simulink model "sgMdl_IO203_DigitalLoopback"  (R2024b)
settings: Solver=FixedStepAuto  StartTime=0.0  StopTime=inf  RelTol=1e-3  EnableMultiTasking=on
libraries: speedgoatlib_IO203 x3
Description:
  | IO203 - Digital Loopback
settings Model: ModifiedByFormat=Speedgoat  Creator=Speedgoat  LastModifiedBy=Speedgoat
settings SolverCC: ConcurrentTasks=on  AlgebraicLoopSolver=TrustRegion  PositivePriorityOrder=on
settings DataIOCC: LimitDataPoints=on  SaveFormat=Array  SignalLoggingSaveFormat=ModelDataLogs  ReturnWorkspaceOutputs=off
settings OptimizationCC: BlockReduction=off  OptimizeBlockIOStorage=off  BufferReuse=off  ReuseModelBlockBuffer=off  GlobalBufferReuse=off  ExpressionFolding=off  ExpressionDepthLimit=2147483647  LocalBlockOutputs=off
settings DebuggingCC: UnderspecifiedInitializationDetection=Classic  MergeDetectMultiDrivingBlocksExec=none  SolverPrmCheckMsg=warning  TasksWithSamePriorityMsg=none  FcnCallInpInsideContextMsg=warning  StateNameClashWarn=warning  SFUnexpectedBacktrackingDiag=warning  SFNoUnconditionalDefaultTransitionDiag=warning  SFExecutionAtInitializationDiag=none  ArithmeticOperatorsInVariantConditions=warning
settings HardwareCC: ProdBitPerLong=64  ProdLongLongMode=on  ProdHWDeviceType=Intel->x86-64 (Linux 64)
settings ModelReferenceCC: EnableRefExpFcnMdlSchedulingChecks=on  PropagateSignalLabelsOutOfModel=off
settings SFSimCC: SimUseLocalCustomCode=off  CustomCodeUndefinedFunction=UseInterfaceOnly
settings RTWCC: Description=Speedgoat Real-Time Target Machine  SystemTargetFile=speedgoat.tlc  TemplateMakefile=slrealtime_default_tmf  RTWUseLocalCustomCode=off  Toolchain=Simulink Real-Time Toolchain  BuildConfiguration=Faster Runs  TargetLang=C++  GPUComputeCapability=3.5  DLArmComputeVersion=19.05
settings CodeAppCC: StateflowObjectComments=on
settings SimulinkRealTimeTargetCC: SubcomponentCodeInterfacePackaging=Reusable function  InstructionSetFMA=off  LogToMDFFile=off  SLRTFileLogMaxRuns=10
settings ConfigComp: CovMetricSettings=dw  CovSaveCumulativeToWorkspaceVar=on  CovSaveSingleToWorkspaceVar=on  CovExternalEMLEnable=off  CovSFcnEnable=off  CovBoundaryAbsTol=1.0e-5

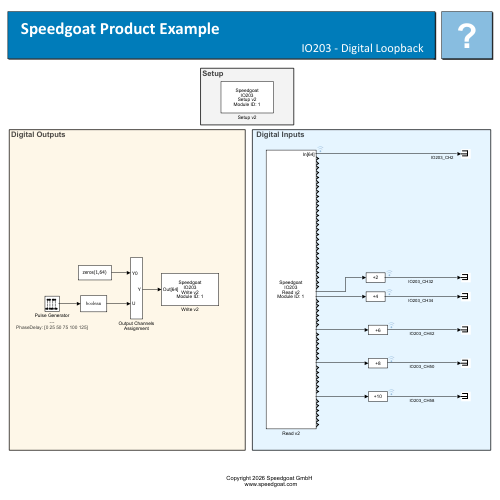
[thumbnail: Simulink's stored preview of the top-level diagram]
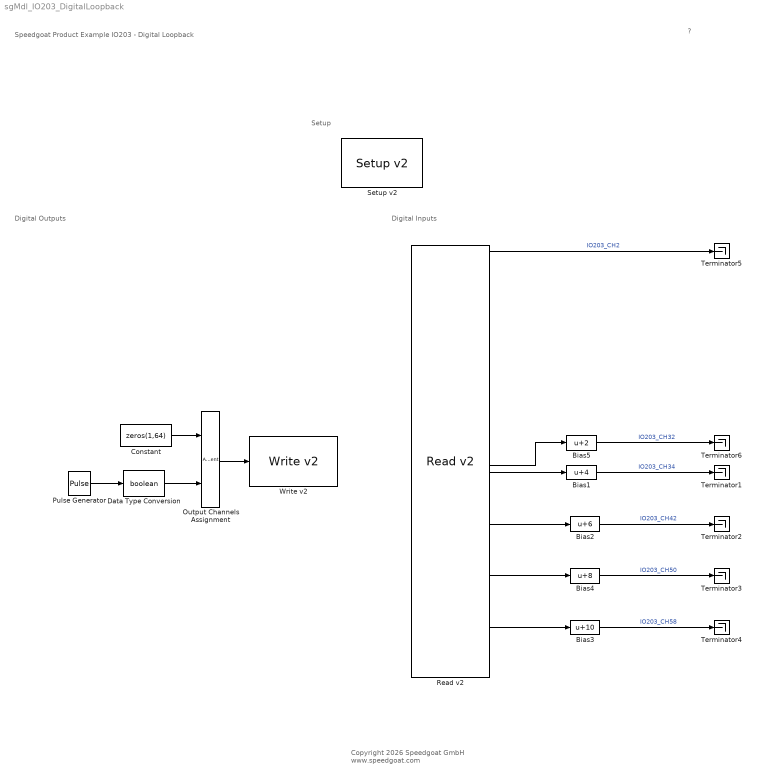
== system sgMdl_IO203_DigitalLoopback ==
  note: Digital Outputs
  note: Setup
  note: Digital Inputs
  note: Speedgoat Product Example
      | IO203 - Digital Loopback
  note: ?
  note: Copyright 2026 Speedgoat GmbH
      |  www.speedgoat.com
  Bias1 : Bias  Bias=4  SaturateOnIntegerOverflow=off
  Bias2 : Bias  Bias=6  SaturateOnIntegerOverflow=off
  Bias3 : Bias  Bias=10  SaturateOnIntegerOverflow=off
  Bias4 : Bias  Bias=8  SaturateOnIntegerOverflow=off
  Bias5 : Bias  Bias=2  SaturateOnIntegerOverflow=off
  Constant : Constant  Value=zeros(1,64)  OutDataTypeStr=boolean  SampleTime=-1
  Data Type Conversion : DataTypeConversion  OutDataTypeStr=boolean  SaturateOnIntegerOverflow=off  RndMeth=Floor
  Output Channels Assignment : Assignment  DiagnosticForDimensions=Warning  IndexOptions=Index vector (dialog)  Indices=[1 31 33 41 49 57]  OutputSizes=1
  Pulse Generator : DiscretePulseGenerator  Period=[100 100 100 200 200 200]  PulseWidth=[50 50 50 100 100 100]  PhaseDelay=[0 25 50 75 100 125]  SampleTime=0.001
      settings: AttributesFormatString=|
      | ---
      | PhaseDelay: %<PhaseDelay>
  Read v2 : speedgoatlib_IO203/Read v2   parId=1  parPortConf=1 port for each active input channel  parDataType=Double  parSampleTime=0.001  readPorts=[2 3 4 5 6 7 8 9 10 11 12 13 14 15 16 17 18 19 20 21 22 23 24 25 26 27 28 29 30 32 34 35 36 37 38 39 40 42 43 44 45 46 47 48 50 51 52 53 54 55 56 58 59 60 61 62 63 64]  portList=[2 3 4 5 6 7 8 9 10 11 12 13 14 15 16 17 18 19 20 21 22 23 24 25 26 27 28 29 30 32 34 35 36 37 38 39 40 42 43 44 45 46 47 48 50 51 52 53 54 55 56 58 59 60 61 62 63 64]  parPciSlot=-1  parNumOfPorts=58
      settings: SourceProductName=IO203
  Setup v2 : speedgoatlib_IO203/Setup v2   parId=1  parPciSlot=-1  parEnableTtl=off  parSelDirMethod=off  parDirVect=[1, 0, zeros(1,28), 1, 0, 1, 0, zeros(1,6), 1, 0, zeros(1,6), 1, 0, zeros(1,6), 1, 0, zeros(1,6)]  visCh1=on  visCh2=off  visCh3=off  visCh4=off  visCh5=off  visCh6=off  visCh7=off  visCh8=off  visCh9=off  visCh10=off  visCh11=off  visCh12=off  visCh13=off  visCh14=off  visCh15=off  visCh16=off  visCh17=off  visCh18=off  visCh19=off  visCh20=off  visCh21=off  visCh22=off  visCh23=off  visCh24=off  visCh25=off  visCh26=off  visCh27=off  visCh28=off  visCh29=off  visCh30=off  visCh31=on  visCh32=off  visCh33=on  visCh34=off  visCh35=off  visCh36=off  visCh37=off  visCh38=off  visCh39=off  visCh40=off  visCh41=on  visCh42=off  visCh43=off  visCh44=off  visCh45=off  visCh46=off  visCh47=off  visCh48=off  visCh49=on  visCh50=off  visCh51=off  visCh52=off  visCh53=off  visCh54=off  visCh55=off  visCh56=off  visCh57=on  visCh58=off  visCh59=off  visCh60=off  visCh61=off  visCh62=off  visCh63=off  visCh64=off  parResetVect=[1]  parInitValVect=[0]
      settings: SourceProductName=IO203
  Terminator{1..6} (6 alike) : Terminator
  Write v2 : speedgoatlib_IO203/Write v2   parId=1  parPortConf=1 port with a 64 elements vector  parSampleTime=-1  writePorts=[1 31 33 41 49 57]  portList=[1 31 33 41 49 57]  parPciSlot=-1  parEnableTtl=off  parNumOfPorts=6
      settings: SourceProductName=IO203
  wires:
  Bias2/1 -> Terminator2/1  "IO203_CH42"
  Bias4/1 -> Terminator3/1  "IO203_CH50"
  Bias1/1 -> Terminator1/1  "IO203_CH34"
  Read v2/1 -> Terminator5/1  "IO203_CH2"
  Bias5/1 -> Terminator6/1  "IO203_CH32"
  Pulse Generator/1 -> Data Type Conversion/1
  Constant/1 -> Output Channels Assignment/1
  Bias3/1 -> Terminator4/1  "IO203_CH58"
  Output Channels Assignment/1 -> Write v2/1
  Read v2/38 -> Bias2/1
  Read v2/45 -> Bias4/1
  Read v2/52 -> Bias3/1
  Read v2/31 -> Bias1/1
  Read v2/30 -> Bias5/1
  Data Type Conversion/1 -> Output Channels Assignment/2
